simulink model "MultirotorSimPx4v1_8RateTuning"  (R2018b)
settings: Solver=VariableStepAuto  StartTime=0.0  StopTime=Simulation.T_END  MaxStep=Simulation.TS_MAX  RelTol=1e-3  EnableMultiTasking=on
PreLoadFcn:
  | % InitializeParameters;
undefined symbols (not defined in the file): Initial, Simulation, Uav
libraries: QuaternionLibrary x13, simulink_extras x10
(part 1 of 7)
settings Model: Creator=jban039  LastModifiedBy=jban039
settings DataIOCC: Decimation=10  ReturnWorkspaceOutputs=on  OutputOption=SpecifiedOutputTimes  OutputTimes=Simulation.T_OUT
settings OptimizationCC: LifeSpan=inf
settings DebuggingCC: ReadBeforeWriteMsg=DisableAll  WriteAfterWriteMsg=DisableAll  WriteAfterReadMsg=DisableAll  MultiTaskDSMMsg=none  UnconnectedLineMsg=none  AllowSymbolicDim=off  SFUnexpectedBacktrackingDiag=warning  SFNoUnconditionalDefaultTransitionDiag=warning  SFExecutionAtInitializationDiag=none  UnderSpecifiedDimensionMsg=warning
settings ModelReferenceCC: UpdateModelReferenceTargets=IfOutOfDate  ModelReferenceMinAlgLoopOccurrences=on  PropagateSignalLabelsOutOfModel=off
settings SFSimCC: SFSimEcho=off  SimUseLocalCustomCode=off
settings RTWCC: RTWUseLocalCustomCode=off
settings CodeAppCC: StateflowObjectComments=on
settings GRTTargetCC: TargetLangStandard=C89/C90 (ANSI)
settings ConfigComp: CovMetricSettings=dw  CovHtmlReporting=on  CovSaveCumulativeToWorkspaceVar=on  CovSaveSingleToWorkspaceVar=on  CovExternalEMLEnable=off

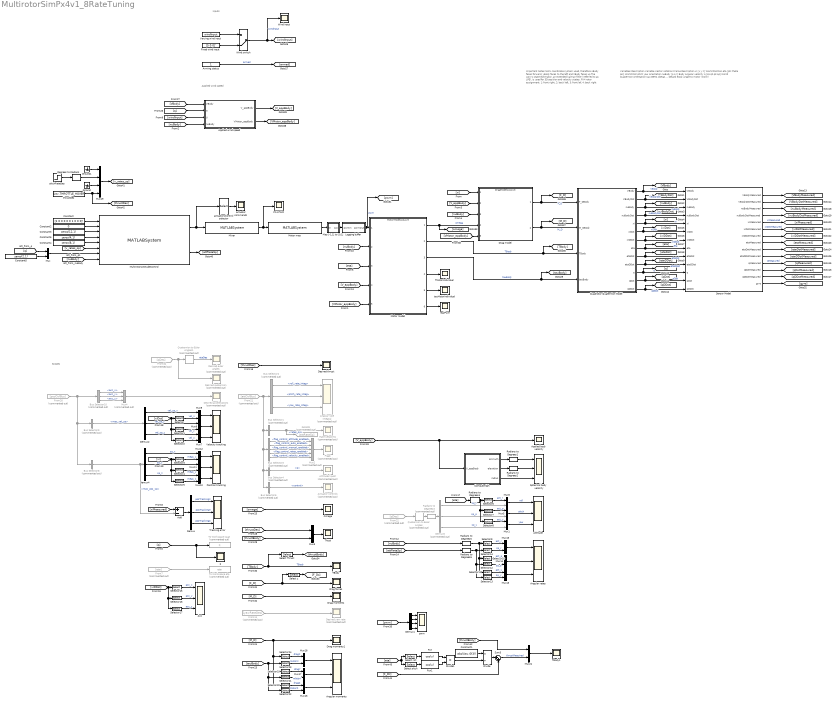
== system MultirotorSimPx4v1_8RateTuning ==
  note: Important Notes
      |
      | NWU coordinate system used, therefore xBody faces forward, yBody faces to the left and zBody faces up
      | The UAV's state estimator, an extended kalman filter (referred to as LPE), is used for 3D position and velocity states.
      | PX4 rotor assignment: 1: front right, 2: back left, 3: front lef, 4: back right
  note: Variables Description
      |
      | Variable
      | Vector notation
      | Frame
      | Description
      |
      | xi
      | [x y z]
      | World
      | Position
      |
      | eta
      | [phi theta psi]
      | World
      | Roll pitch yaw orientation
      |
      | nuBody
      | [p q r]
      | Body
      | Angular velocity
      |
      | q
      | [q1 q2 q3 q4]
      | World
      | Quaternion orientation
      |
      | Uav.BETA
      | [beta1 ... betaN]
      | Body
      | Angle to motor (CCW)
  note: Applied wind speed
  note: Inputs
  note: Scopes
  Acc : Scope  NumInputPorts=3
  Actuator controls : Scope  Commented=on
  Add : Sum  Inputs=+-
  Angular moments : Scope  NumInputPorts=3
  Angular rate integral : Scope  Commented=on  NumInputPorts=3
  Angular rates : Scope  NumInputPorts=3
  Applied body velocity : Scope
  Applied wind speed : Subsystem
  Arming status : Constant
  Attitude : Scope  NumInputPorts=3
  Attitude (quat) : Scope  Commented=on
  Bus Selector1 : BusSelector  Commented=on  OutputSignals=rates_sp
  Bus Selector10 : BusSelector  Commented=on  OutputSignals=mpc_local_pos_sp.acc_x,mpc_local_pos_sp.acc_y,mpc_local_pos_sp.acc_z
  Bus Selector2 : BusSelector  Commented=on  OutputSignals=controller_status.roll_rate_integ,controller_status.pitch_rate_integ,controller_status.yaw_rate_integ
  Bus Selector3 : BusSelector  Commented=on  OutputSignals=v_control_mode.flag_control_attitude_enabled,v_control_mode.flag_control_auto_enabled,v_control_mode.flag_control_manual_enabled,v_control_mode.flag_control_rates_enabled,v_control_mode.flag_control_velocity_enabled
  Bus Selector4 : BusSelector  Commented=on  OutputSignals=ctrl_state.q
  Bus Selector6 : BusSelector  Commented=on  OutputSignals=actuators.control
  Bus Selector8 : BusSelector  Commented=on  OutputSignals=mpc_pos_sp
  Bus Selector9 : BusSelector  Commented=on  OutputSignals=mpc_vel_sp
  Compute Sph : MATLAB Function  TreatAsAtomicUnit=on
  Constant : Constant  Value=[1 0 0 0 0 0 1 0 0 0]'
  Constant1 : Constant  Value=abs(Uav.G(3))
  Constant2 : Constant  Value=0
  Constant3 : Constant  Value=zeros(12,1)
  Constant4 : Constant  Value=zeros(8,1)
  Constant5 : Constant  Value=zeros(2,1)
  Constant6 : Constant  Value=zeros(4,1)
  Degrees to Radians : simulink_extras/Transformations/Degrees to Radians
  Demux : Demux  Outputs=3
  Demux1 : Demux
  Demux2 : Demux  Outputs=3
  Demux4 : Demux  Outputs=3
  Demux6 : Demux  Commented=on  Outputs=3
  Desired accelerations : Scope  Commented=on
  Desired euler angles : Scope  Commented=on
  Desired quaternion : Scope  Commented=on
  Desired thrust : Scope
  Desired yaw rate : Scope  Commented=on
  Divide : Product  Inputs=*/
  Divide1 : Product  Inputs=**
  Drag forces : Scope
  Drag model : ModelReference  ModelNameDialog=DragModelAIAAv3  SimulationMode=Normal  ModelReferenceVersion=1.368
  Drag moments : Scope
  Drag moments1 : Scope
  Fcn : Fcn  Expr=cos(u)
  Fcn1 : Fcn  Expr=cos(u)
  Fixed wind input : Constant  Value=[5 0 0]'
  Flags : Scope  Commented=on
  From11 : From  Commented=on  GotoTag=yawRateDes
  From20 : From  Commented=on  GotoTag=posCtrlBus
  From21 : From  Commented=on  GotoTag=attCtrlBus
  From22 : From  Commented=on  GotoTag=qDes
  From34 : From  Commented=on  GotoTag=qDes
  From7 : From  Commented=on  GotoTag=eta
  Goto28 : Goto  Commented=on  GotoTag=attRateSp
  Ground : Ground
  Ground1 : Ground
  Logging buffer : Subsystem
  Map [-1,1] to [0,1] : Subsystem
  Mixer : MATLABSystem  System=MultirotorMixer  airframeConfig=5  useHorThrust=0  outputSatStatus=0  SimulateUsing=Code generation
      mask Type: MultirotorMixer
      mask Display:
      | disp(['MULTIROTOR' char(10) 'MIXER' char(10) 'octa_x']);
      | port_label('input',1,'actuatorsControl');
      | port_label('output',1,'px4PWM');
  Motor map : MATLABSystem  System=MotorMap  airframeConfig=5  SimulateUsing=Code generation
      mask Type: MotorMap
      mask Display:
      | disp(['MOTOR' char(10) 'MAP' char(10) 'octa_x']);
      | port_label('input',1,'px4PWM');
      | port_label('output',1,'simPWM');
  Motor model : ModelReference  ModelNameDialog=MotorModelAIAAv3  SimulationMode=Normal  ModelReferenceVersion=1.397
  MultirotorAttitudeControl : MATLABSystem  System=MulticopterAttitudeControl  acro_expo_rp=0.69  acro_expo_y=0.69  acro_pitch_max=720  acro_roll_max=720  acro_superexpo_rp=0.7  acro_superexpo_y=0.7  acro_yaw_max=540  airmode=0  d_term_cutoff_freq=30  pitch_rate_d=0.003  pitch_rate_ff=0  pitch_rate_i=0.05  pitch_rate_max=220  pitch_rate_p=0.15  pitch_p=6.5  pitch_rate_integ_lim=0.3  rattitude_thres=0.8  roll_rate_d=0.003  roll_rate_ff=0  roll_rate_i=0.05  roll_rate_max=220  roll_rate_p=0.15  roll_p=6.5  roll_rate_integ_lim=0.3  tpa_breakpoint_d=1  tpa_breakpoint_i=1  tpa_breakpoint_p=1  tpa_rate_d=0  tpa_rate_i=0  tpa_rate_p=0  yaw_rate_d=0  yaw_rate_ff=0  yaw_rate_i=0.1  yaw_rate_max=200  yaw_rate_p=0.2  yaw_auto_max=45  yaw_p=2.8  yaw_rate_integ_lim=0.3  man_throttle_min=0.08  man_tilt_max_deg=35  yaw_rate_scaling=200  throttle_hover=0.5  throttle_max=1  board_rotation_param=0  board_offset_x=0  board_offset_y=0  board_offset_z=0  bat_scale_en=0  throttle_curve=0  vehicle_status_is_rotary_wing=1  vehicle_status_is_vtol=0  loop_update_rate_hz=250  simple_mode=0  output_rates=1  SimulateUsing=Code generation
      mask Type: MulticopterAttitudeControl
      mask Display:
      | disp(['MulticopterAttitudeControl' char(10) '' char(10) 'v1.82']);
      | port_label('input',1,'v_control_mode_flags');
      | port_label('input',2,'vehicle_land_detected');
      | port_label('input',3,'saturation_status');
      | port_label('input',4,'manual_control_sp');
      | port_label('input',5,'v_att_sp');
      | port_label('input',6,'v_rates_sp');
      | port_label('input',7,'v_att_in');
      | port_label('input',8,'sensor_gyro');
      | port_label('output',1,'actuatorsControl');
      | port_label('output',2,'attRateSp');
  Mux{,1,3,5..18,21} (18 alike) : Mux  Inputs=2
  Mux19 : Mux
  Mux2 : Mux  Commented=on  Inputs=5
  Mux4 : Mux  Commented=on  Inputs=3
  Omega : Scope
  PX4 PWM : Scope
  Position tracking : Scope  NumInputPorts=3
  Quadrotor Quaternion Model : Subsystem
  Quaternion to Euler Angles : QuaternionLibrary/Quaternion to Euler Angles  Commented=on
  Quaternion to Euler Angles1 : QuaternionLibrary/Quaternion to Euler Angles  Commented=on
  Radians to Degrees{1..2,4..6} (5 alike) : simulink_extras/Transformations/Radians to Degrees
  Radians to Degrees3 : simulink_extras/Transformations/Radians to Degrees  Commented=on
  Rate setpoints : Scope  Commented=on
  Select Thrust : Selector  InputPortWidth=3  IndexOptions=Index vector (dialog)  Indices=[3]  OutputSizes=1
  Select pitch : Selector  InputPortWidth=3  IndexOptions=Index vector (dialog)  Indices=2  OutputSizes=1
  Select roll : Selector  InputPortWidth=3  IndexOptions=Index vector (dialog)  Indices=1  OutputSizes=1
  Select z : Selector  InputPortWidth=3  IndexOptions=Index vector (dialog)  Indices=[3]  OutputSizes=1
  Selector{,3,6,9,14..15,23..24} (8 alike) : Selector  InputPortWidth=3  IndexOptions=Index vector (dialog)  Indices=1  OutputSizes=1
  Selector{1,4,7,10,12,16,19,21} (8 alike) : Selector  InputPortWidth=3  IndexOptions=Index vector (dialog)  Indices=2  OutputSizes=1
  Selector{2,5,8,11,13,17,20,22} (8 alike) : Selector  InputPortWidth=3  IndexOptions=Index vector (dialog)  Indices=3  OutputSizes=1
  Sensor Model : Subsystem
  Spherical body velocity : Scope  NumInputPorts=3
  Sum3 : Sum  Inputs=|++
  TBody : Scope
  TBody1 : Scope
  TMotorIndividual : Scope
  Thust : Scope
  To Workspace eta : ToWorkspace  Commented=on  VariableName=eta  SaveFormat=Structure With Time  SampleTime=0.01
  To Workspace quat : ToWorkspace  Commented=on  VariableName=q  SaveFormat=Structure With Time  SampleTime=0.01
  Tracking error : Scope  NumInputPorts=3
  Varying wind input : FromWorkspace  VariableName=windInput  SampleTime=0
  Velocity tracking : Scope  NumInputPorts=3
  Wind Input : Scope
  Wind switch : ManualSwitch  CurrentSetting=0
  actuator commands : Scope
  actuatorsControl selector : Selector  InputPortWidth=8  IndexOptions=Index vector (dialog)  Indices=[1 2 3]  OutputSizes=1
  pitchRateDes : Step  After=30  SampleTime=0
  pwm : Scope  NumInputPorts=4
  q : Scope
  realPwm : Scope
  tauMotorIndividual : Scope
  thrustDes : Constant  Value=Uav.THROTTLE_HOVER
  wires:
  Motor model/1 -> [omega], Drag model/4  "omega"
  Motor model/2 -> Quadrotor Quaternion Model/3(TBody), [TBody]  "TBody"
  Drag model/2 -> Quadrotor Quaternion Model/2(M_DBody), [M_D]  "M_D"
  Quadrotor Quaternion Model/1(VBody) -> Sensor Model/1(VBody), [VBody]  "VBody"
  Quadrotor Quaternion Model/2(VBodyDot) -> Sensor Model/2(VBodyDot), [VBodyDot]  "VBodyDot"
  Quadrotor Quaternion Model/3(nuBody) -> Sensor Model/3(nuBody), [nuBody]  "nuBody"
  Quadrotor Quaternion Model/4(nuBodyDot) -> Sensor Model/4(nuBodyDot), [nuBodyDot]  "nuBodyDot"
  Quadrotor Quaternion Model/5(xi) -> Sensor Model/5(xi), [xi]  "xi"
  Quadrotor Quaternion Model/6(xiDot) -> Sensor Model/6(xiDot), [xiDot]  "xiDot"
  Quadrotor Quaternion Model/7(xiDDot) -> Sensor Model/7(xiDDot), [xiDDot]  "xiDDot"
  Quadrotor Quaternion Model/8(eta) -> Sensor Model/8(eta), [eta]  "eta"
  Quadrotor Quaternion Model/9(etaDot) -> Sensor Model/9(etaDot), [etaDot]  "etaDot"
  Quadrotor Quaternion Model/10(etaDDot) -> Sensor Model/10(etaDDot), [etaDDot]  "etaDDot"
  [V_appBody] -> Drag model/2
  [nuBody] -> Motor model/2
  Quadrotor Quaternion Model/11(q) -> Sensor Model/11(q), [q]  "q"
  Quadrotor Quaternion Model/12(qDot) -> Sensor Model/12(qDot), [qDot]  "qDot"
  Quadrotor Quaternion Model/13(qDDot) -> Sensor Model/13(qDDot), [qDDot]  "qDDot"
  Drag model/1 -> Quadrotor Quaternion Model/1(F_DBody), [F_D]  "F_D"
  Sensor Model/1(VBodyMeasured) -> [VBodyMeasured]
  Sensor Model/2(VBodyDotMeasured) -> [VBodyDotMeasured]
  Sensor Model/3(nuBodyMeasured) -> [nuBodyMeasured]
  Sensor Model/4(nuBodyDotMeasured) -> [nuBodyDotMeasured]
  Sensor Model/5(xiMeasured) -> [xiMeasured]  "xiMeasured"
  Sensor Model/6(xiDotMeasured) -> [xiDotMeasured]  "xiDotMeasured"
  Sensor Model/7(xiDDotMeasured) -> [xiDDotMeasured]
  Sensor Model/8(etaMeasured) -> [etaMeasured]
  Sensor Model/9(etaDotMeasured) -> [etaDotMeasured]
  Sensor Model/10(etaDDotMeasured) -> [etaDDotMeasured]
  Sensor Model/11(qMeasured) -> [qMeasured]  "qMeasured"
  Sensor Model/12(qDotMeasured) -> [qDotMeasured]
  Sensor Model/13(qDDotMeasured) -> [qDDotMeasured]
  Logging buffer/1(pwmOut) -> [pwm], Motor model/1  "pwm"
  Bus Selector2/1 -> Angular rate integral/1  "<roll_rate_integ>"
  Bus Selector2/2 -> Angular rate integral/2  "<pitch_rate_integ>"
  Bus Selector2/3 -> Angular rate integral/3  "<yaw_rate_integ>"
  From21/1 -> Bus Selector2/1, Bus Selector1/1, Bus Selector6/1, Bus Selector4/1, Bus Selector3/1
  Bus Selector1/1 -> Goto28/1, Rate setpoints/1  "<rates_sp>"
  Bus Selector3/1 -> Mux2/1  "<flag_control_attitude_enabled>"
  Bus Selector3/2 -> Mux2/2  "<flag_control_auto_enabled>"
  Bus Selector3/3 -> Mux2/3  "<flag_control_manual_enabled>"
  Bus Selector3/4 -> Mux2/4  "<flag_control_rates_enabled>"
  Bus Selector3/5 -> Mux2/5  "<flag_control_velocity_enabled>"
  Mux2/1 -> Flags/1
  Bus Selector4/1 -> Attitude (quat)/1  "<q>"
  Bus Selector6/1 -> Actuator controls/1  "<control>"
  From20/1 -> Bus Selector10/1, Bus Selector9/1, Bus Selector8/1
  [q] -> Mux/1
  Bus Selector9/1 -> Demux2/1  "<mpc_vel_sp>"
  Bus Selector10/1 -> Mux4/1  "<acc_x>"
  Bus Selector10/2 -> Mux4/2  "<acc_y>"
  Bus Selector10/3 -> Mux4/3  "<acc_z>"
  Mux4/1 -> Desired accelerations/1
  Selector6/1 -> Mux6/1  "act_r"
  Selector7/1 -> Mux5/1  "act_p"
  Mux7/1 -> Velocity tracking/3
  Mux8/1 -> Velocity tracking/2
  Mux9/1 -> Velocity tracking/1
  Demux2/1 -> Mux9/1  "vel_sp_x"
  Selector/1 -> Mux9/2  "vel_x"
  Demux2/2 -> Mux8/1  "vel_sp_y"
  Selector1/1 -> Mux8/2  "vel_y"
  Demux2/3 -> Mux7/1  "vel_sp_z"
  Selector2/1 -> Mux7/2  "vel_z"
  Mux10/1 -> Position tracking/3
  Mux11/1 -> Position tracking/2
  Mux12/1 -> Position tracking/1
  Demux4/1 -> Mux12/1  "sp_x"
  Selector3/1 -> Mux12/2  "meas_x"
  Demux4/2 -> Mux11/1  "sp_y"
  Selector4/1 -> Mux11/2  "meas_y"
  Demux4/3 -> Mux10/1  "sp_z"
  Selector5/1 -> Mux10/2  "meas_z"
  Quaternion to Euler Angles/1 -> Radians to Degrees3/1
  Demux6/1 -> Mux6/2  "sp_r"
  Demux6/2 -> Mux5/2  "sp_p"
  Demux6/3 -> Mux1/2  "sp_y"
  Selector8/1 -> Mux1/1  "act_y"
  From22/1 -> Quaternion to Euler Angles/1
  Mixer/1 -> Motor map/1, PX4 PWM/1
  Bus Selector8/1 -> Add/2, Demux4/1  "<mpc_pos_sp>"
  Add/1 -> Demux/1
  Demux/1 -> Tracking error/1  "posTrackingX"
  Demux/2 -> Tracking error/2  "posTrackingY"
  Demux/3 -> Tracking error/3  "posTrackingZ"
  [nuBody] -> Drag model/3
  Mux6/1 -> Attitude/1  "roll"
  Mux5/1 -> Attitude/2  "pitch"
  [eta] -> Motor model/3
  [q] -> q/1, To Workspace quat/1
  From7/1 -> To Workspace eta/1
  [xiDot] -> Selector2/1, Selector1/1, Selector/1
  [xi] -> Selector5/1, Selector4/1, Selector3/1
  [xiMeasured] -> Add/1
  Wind switch/1 -> [windInput], Wind Input/1  "windInput"
  [V_appBody] -> Motor model/4
  Arming status/1 -> [armed]  "armed"
  Fixed wind input/1 -> Wind switch/2
  Varying wind input/1 -> Wind switch/1
  [omega] -> Omega/1
  Radians to Degrees3/1 -> Demux6/1
  Radians to Degrees4/1 -> Selector8/1, Selector7/1, Selector6/1
  [eta] -> Radians to Degrees4/1
  Motor model/4 -> TMotorIndividual/1
  [thrustDes] -> Mux3/1
  [thrustBody] -> Mux3/2
  Mux3/1 -> Thust/1
  Motor model/5 -> tauMotorIndividual/1
  [xi] -> Drag model/1
  [TBody] -> Select Thrust/1, TBody/1  "TBody"
  Select Thrust/1 -> [thrustBody]
  [F_D] -> Drag forces/1, Select z/1
  [V_appBody] -> Compute Sph/1(V_appBody), Applied body velocity/1
  Compute Sph/1(azimuth) -> Radians to Degrees1/1
  Compute Sph/2(elevation) -> Radians to Degrees2/1
  Compute Sph/3(radius) -> Spherical body velocity/3
  Radians to Degrees1/1 -> Spherical body velocity/1
  Radians to Degrees2/1 -> Spherical body velocity/2
  [M_D] -> Drag moments/1
  [VMotor_appBody] -> Motor model/5
  [VMotor_appBody] -> Drag model/5
  From11/1 -> Desired yaw rate/1
  Mux1/1 -> Attitude/3  "yaw"
  Motor model/3 -> Quadrotor Quaternion Model/4(tauBody), [tauBody]  "tauBody"
  [VBody] -> Applied wind speed/1(VBody)
  [q] -> Applied wind speed/2(q)
  [windInput] -> Applied wind speed/3(U)
  Applied wind speed/1(V_appBody) -> [V_appBody]
  Applied wind speed/2(VMotor_appBody) -> [VMotor_appBody]
  [nuBody] -> Applied wind speed/4(nuBody)
  Selector9/1 -> Mux15/1  "act_r"
  Selector10/1 -> Mux14/1  "act_p"
  Selector11/1 -> Mux13/1  "act_y"
  Mux15/1 -> Angular rates/1
  Mux14/1 -> Angular rates/2
  Radians to Degrees5/1 -> Selector9/1, Selector11/1, Selector10/1
  [nuBody] -> Radians to Degrees5/1
  Mux13/1 -> Angular rates/3
  Radians to Degrees6/1 -> Selector14/1, Selector13/1, Selector12/1
  Selector14/1 -> Mux15/2  "sp_r"
  Selector12/1 -> Mux14/2  "sp_p"
  Selector13/1 -> Mux13/2  "sp_y"
  [attRateSp] -> Radians to Degrees6/1
  Selector15/1 -> Acc/1  "acc_x"
  Selector16/1 -> Acc/2  "acc_y"
  Selector17/1 -> Acc/3  "acc_z"
  [xiDDot] -> Selector15/1, Selector16/1, Selector17/1
  [thrustDes] -> Desired thrust/1
  actuatorsControl selector/1 -> actuator commands/1
  [M_D] -> Selector20/1, Selector19/1, Selector24/1, Drag moments1/1
  Mux18/1 -> Angular moments/1
  Mux17/1 -> Angular moments/2
  Mux16/1 -> Angular moments/3
  Selector24/1 -> Mux18/1  "dragX"
  Selector23/1 -> Mux18/2  "motorX"
  Selector19/1 -> Mux17/1  "dragY"
  Selector21/1 -> Mux17/2  "motorY"
  Selector20/1 -> Mux16/1  "dragZ"
  Selector22/1 -> Mux16/2  "MotorZ"
  [tauBody] -> Selector22/1, Selector21/1, Selector23/1
  From34/1 -> Desired quaternion/1, Quaternion to Euler Angles1/1
  Quaternion to Euler Angles1/1 -> Desired euler angles/1  "etaDes"
  Divide/1 -> Sum3/1
  Sum3/1 -> Mux21/2  "thrustRequired"
  Mux21/1 -> TBody1/1
  Constant1/1 -> Divide/1
  Select z/1 -> [F_Dz]
  [thrustBody] -> Mux21/1
  [eta] -> Select pitch/1, Select roll/1
  Select roll/1 -> Fcn/1
  Select pitch/1 -> Fcn1/1
  Fcn/1 -> Divide1/1
  Fcn1/1 -> Divide1/2
  Divide1/1 -> Divide/2
  [F_Dz] -> Sum3/2
  [pwm] -> Demux1/1
  Demux1/1 -> pwm/1
  Demux1/2 -> pwm/2
  Demux1/3 -> pwm/3
  Demux1/4 -> pwm/4
  Motor model/6 -> realPwm/1
  Sensor Model/14(gyro) -> [gyro]
  [nuBody] -> MultirotorAttitudeControl/8
  MultirotorAttitudeControl/2 -> [attRateSp]
  Motor map/1 -> Map [-1,1] to [0,1]/1(in)
  Map [-1,1] to [0,1]/1(out) -> Logging buffer/1(pwmIn)
  MultirotorAttitudeControl/1 -> Mixer/1, actuatorsControl selector/1
  Constant/1 -> MultirotorAttitudeControl/1
  Constant2/1 -> MultirotorAttitudeControl/2
  Constant3/1 -> MultirotorAttitudeControl/3
  Constant4/1 -> MultirotorAttitudeControl/5
  Constant5/1 -> Mux/2
  Mux/1 -> MultirotorAttitudeControl/7
  Constant6/1 -> MultirotorAttitudeControl/4
  [v_rates_sp] -> MultirotorAttitudeControl/6
  Mux19/1 -> [v_rates_sp]
  pitchRateDes/1 -> Degrees to Radians/1
  Ground/1 -> Mux19/3
  thrustDes/1 -> [thrustDes], Mux19/4
  Ground1/1 -> Mux19/1
  Degrees to Radians/1 -> Mux19/2

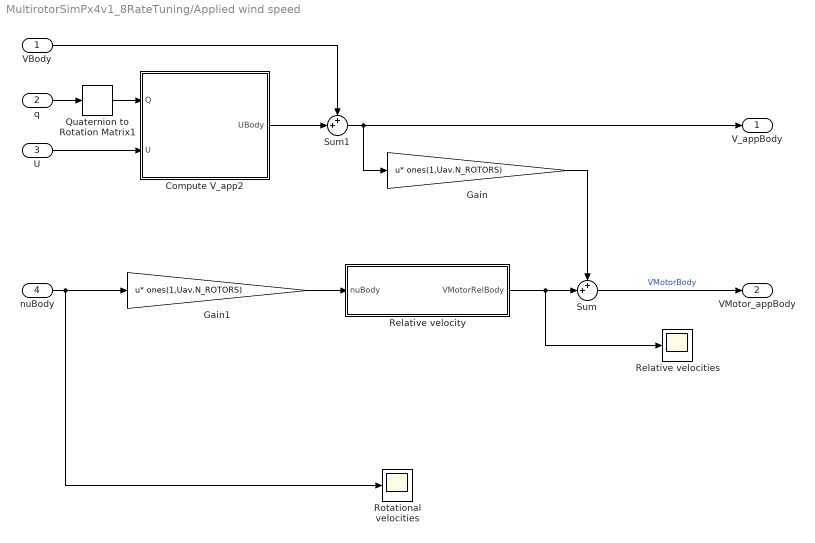
== system MultirotorSimPx4v1_8RateTuning/Applied wind speed ==
  VBody : Inport  Unit=m/s
  q : Inport  Port=2
  U : Inport  Port=3  Unit=m/s
  nuBody : Inport  Port=4  Unit=rad/s
  Compute V_app2 : MATLAB Function  TreatAsAtomicUnit=on
  Gain : Gain  Gain=ones(1,Uav.N_ROTORS)  Multiplication=Matrix(u*K)
  Gain1 : Gain  Gain=ones(1,Uav.N_ROTORS)  Multiplication=Matrix(u*K)
  Quaternion to Rotation Matrix1 : QuaternionLibrary/Quaternion to Rotation Matrix
  Relative velocities : Scope
  Relative velocity : MATLAB Function  TreatAsAtomicUnit=on
  Rotational velocities : Scope
  Sum : Sum  Inputs=++|
  Sum1 : Sum  Inputs=++|
  V_appBody : Outport  Unit=m/s
  VMotor_appBody : Outport  Port=2  Unit=m/s  PortDimensions=[3,Uav.N_ROTORS]
  wires:
  U/1 -> Compute V_app2/2(U)
  Sum/1 -> VMotor_appBody/1  "VMotorBody"
  Quaternion to Rotation Matrix1/1 -> Compute V_app2/1(Q)
  nuBody/1 -> Gain1/1, Rotational velocities/1
  Gain/1 -> Sum/1
  VBody/1 -> Sum1/1
  q/1 -> Quaternion to Rotation Matrix1/1
  Relative velocity/1(VMotorRelBody) -> Relative velocities/1, Sum/2
  Compute V_app2/1(UBody) -> Sum1/2
  Sum1/1 -> Gain/1, V_appBody/1
  Gain1/1 -> Relative velocity/1(nuBody)

== system MultirotorSimPx4v1_8RateTuning/Logging buffer ==
  pwmIn : Inport
  Rate Transition : RateTransition
  pwmOut : Outport
  wires:
  pwmIn/1 -> Rate Transition/1
  Rate Transition/1 -> pwmOut/1

== system MultirotorSimPx4v1_8RateTuning/Map [-1,1] to [0,1] ==
  in : Inport
  Constant : Constant
  Gain4 : Gain  Gain=0.5
  Sum : Sum  Inputs=++|
  out : Outport
  wires:
  Sum/1 -> Gain4/1
  Gain4/1 -> out/1
  in/1 -> Sum/2
  Constant/1 -> Sum/1

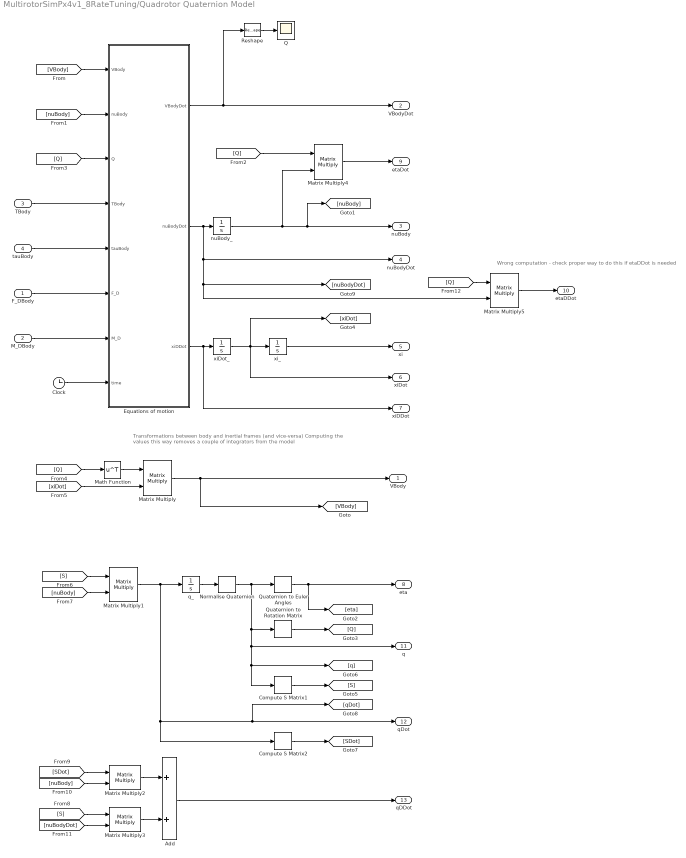
== system MultirotorSimPx4v1_8RateTuning/Quadrotor Quaternion Model ==
  note: Wrong computation - check proper way to do this if etaDDot is needed
  note: Transformations between body and inertial frames (and vice-versa)
      | Computing the values this way removes a couple of integrators from the model
  F_DBody : Inport  Unit=N
  M_DBody : Inport  Port=2  Unit=N*m
  TBody : Inport  Port=3  Unit=N
  tauBody : Inport  Port=4  Unit=N*m
  Add : Sum
  Clock : Clock
  Compute S Matrix1 : QuaternionLibrary/Compute S Matrix
  Compute S Matrix2 : QuaternionLibrary/Compute S Matrix
  Equations of motion : MATLAB Function  TreatAsAtomicUnit=on
  Math Function : Math  Operator=transpose  SaturateOnIntegerOverflow=on
  Matrix Multiply{,1..5} (6 alike) : Product  Multiplication=Matrix(*)
  Normalise Quaternion : QuaternionLibrary/Normalise Quaternion
  Q : Scope
  Quaternion to Euler Angles : QuaternionLibrary/Quaternion to Euler Angles
  Quaternion to Rotation Matrix : QuaternionLibrary/Quaternion to Rotation Matrix
  Reshape : Reshape  OutputDimensionality=Column vector (2-D)
  nuBody_ : Integrator  InitialCondition=Initial.NU_BODY  ContinuousStateAttributes='nuBody'
  q_ : Integrator  InitialCondition=Initial.Q  ContinuousStateAttributes='q'
  xiDot_ : Integrator  InitialCondition=Initial.XI_DOT  ContinuousStateAttributes='xiDot'
  xi_ : Integrator  InitialCondition=Initial.XI  ContinuousStateAttributes='xi'
  VBody : Outport  Unit=m/s
  VBodyDot : Outport  Port=2  Unit=m/s^2
  nuBody : Outport  Port=3  Unit=rad/s
  nuBodyDot : Outport  Port=4  Unit=rad/s^2
  xi : Outport  Port=5  Unit=m
  xiDot : Outport  Port=6  Unit=m/s
  xiDDot : Outport  Port=7  Unit=m/s^2
  eta : Outport  Port=8  Unit=rad
  etaDot : Outport  Port=9  Unit=rad/s
  etaDDot : Outport  Port=10  Unit=rad/s^2
  q : Outport  Port=11
  qDot : Outport  Port=12
  qDDot : Outport  Port=13
  wires:
  Equations of motion/1(VBodyDot) -> Reshape/1, VBodyDot/1
  xi_/1 -> xi/1
  [nuBody] -> Equations of motion/2(nuBody)
  [VBody] -> Equations of motion/1(VBody)
  tauBody/1 -> Equations of motion/5(tauBody)
  TBody/1 -> Equations of motion/4(TBody)
  Equations of motion/3(xiDDot) -> xiDot_/1, xiDDot/1
  F_DBody/1 -> Equations of motion/6(F_D)
  Matrix Multiply/1 -> VBody/1, [VBody]
  M_DBody/1 -> Equations of motion/7(M_D)
  nuBody_/1 -> Matrix Multiply4/2, [nuBody], nuBody/1
  Equations of motion/2(nuBodyDot) -> nuBody_/1, nuBodyDot/1, Matrix Multiply5/2, [nuBodyDot]
  q_/1 -> Normalise Quaternion/1
  Quaternion to Euler Angles/1 -> eta/1, [eta]
  Matrix Multiply4/1 -> etaDot/1
  Quaternion to Rotation Matrix/1 -> [Q]
  [Q] -> Equations of motion/3(Q)
  [Q] -> Math Function/1
  [xiDot] -> Matrix Multiply/2
  Math Function/1 -> Matrix Multiply/1
  [S] -> Matrix Multiply1/1
  [nuBody] -> Matrix Multiply1/2
  Compute S Matrix2/1 -> [SDot]
  [S] -> Matrix Multiply3/1
  Matrix Multiply1/1 -> qDot/1, [qDot], Compute S Matrix2/1, q_/1
  [SDot] -> Matrix Multiply2/1
  [nuBody] -> Matrix Multiply2/2
  [nuBodyDot] -> Matrix Multiply3/2
  Matrix Multiply2/1 -> Add/1
  Matrix Multiply3/1 -> Add/2
  Normalise Quaternion/1 -> Quaternion to Euler Angles/1, q/1, Compute S Matrix1/1, [q], Quaternion to Rotation Matrix/1
  Compute S Matrix1/1 -> [S]
  [Q] -> Matrix Multiply4/1
  Add/1 -> qDDot/1
  [Q] -> Matrix Multiply5/1
  Matrix Multiply5/1 -> etaDDot/1
  Reshape/1 -> Q/1
  xiDot_/1 -> xi_/1, [xiDot], xiDot/1
  Clock/1 -> Equations of motion/8(time)

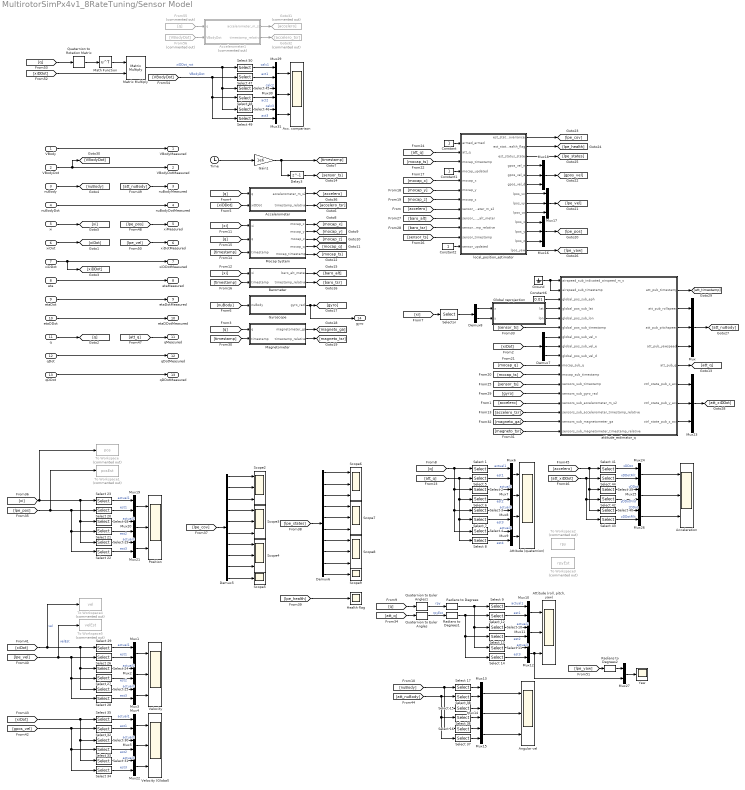
== system MultirotorSimPx4v1_8RateTuning/Sensor Model ==
  VBody : Inport  Unit=m/s  PortDimensions=3
  VBodyDot : Inport  Port=2  Unit=m/s^2  PortDimensions=3
  nuBody : Inport  Port=3  Unit=rad/s  PortDimensions=3
  nuBodyDot : Inport  Port=4  Unit=rad/s^2  PortDimensions=3
  xi : Inport  Port=5  Unit=m  PortDimensions=3
  xiDot : Inport  Port=6  Unit=m/s  PortDimensions=3
  xiDDot : Inport  Port=7  Unit=m/s^2  PortDimensions=3
  eta : Inport  Port=8  Unit=rad  PortDimensions=3
  etaDot : Inport  Port=9  Unit=rad/s  PortDimensions=3
  etaDDot : Inport  Port=10  Unit=rad/s^2  PortDimensions=3
  q : Inport  Port=11  PortDimensions=4
  qDot : Inport  Port=12  PortDimensions=4
  qDDot : Inport  Port=13  PortDimensions=4
  Acc. comparison : Scope  NumInputPorts=3
  Acceleration : Scope  NumInputPorts=3
  Accelerometer : Subsystem
  Accelerometer1 : Subsystem  Commented=on
  Angular vel : Scope  NumInputPorts=3
  Attitude (quaternion) : Scope  NumInputPorts=4
  "Attitude (roll, pitch, yaw)" : Scope  NumInputPorts=3
  Barometer : Subsystem
  Constant : Constant
  Constant1 : Constant
  Constant2 : Constant
  Constant6 : Constant  Value=0.01
  Delay3 : Delay  DelayLength=1  SampleTime=1/400  StateName=sensorTs
  Demux5 : Demux  Outputs=10
  Demux6 : Demux  Outputs=10
  Demux7 : Demux  Outputs=3
  Demux8 : Demux  Outputs=2
  From55 : From  Commented=on  GotoTag=q
  From56 : From  Commented=on  GotoTag=VBodyDot
  Gain1 : Gain  Gain=1e6
  Global reprojection : Subsystem  AncestorBlock=Px4Library/Global reprojection  mask{LAT0=-36.865577, LON0=174.772065}
      mask prompts: LAT0 "Latitude at [x,y] = [0,0]"; LON0 "Longitude at [x,y] = [0,0]"
      mask Display:
      | disp('REPROJECT')
      | port_label('input', 1, sprintf('x'))
      | port_label('input', 2, sprintf('y'))
      | port_label('output', 1, sprintf('lat'))
      | port_label('output', 2, sprintf('lon'))
  Goto31 : Goto  Commented=on  GotoTag=accelero
  Goto32 : Goto  Commented=on  GotoTag=accelero_tsr
  Ground : Ground
  Gyroscope : Subsystem
  Health flag : Scope
  Magnetometer : Subsystem
  Math Function : Math  Operator=transpose  SaturateOnIntegerOverflow=on
  Matrix Multiply : Product  Multiplication=Matrix(*)
  Mocap System : Subsystem
  Mux{,16..18,23} (5 alike) : Mux  Inputs=3
  Mux{1..15,19..22,24..27,29..31} (26 alike) : Mux  Inputs=2
  Position : Scope  NumInputPorts=3
  Quaternion to Euler Angles : QuaternionLibrary/Quaternion to Euler Angles
  Quaternion to Euler Angles1 : QuaternionLibrary/Quaternion to Euler Angles
  Quaternion to Rotation Matrix : QuaternionLibrary/Quaternion to Rotation Matrix
  Radians to Degrees : simulink_extras/Transformations/Radians to Degrees
  Radians to Degrees1 : simulink_extras/Transformations/Radians to Degrees
  Radians to Degrees2 : simulink_extras/Transformations/Radians to Degrees
  Scope{2..4,6..8} (6 alike) : Scope  NumInputPorts=3
  Scope5 : Scope
  Scope9 : Scope
  Select 1 : Selector  InputPortWidth=4  IndexOptions=Index vector (dialog)  Indices=1  OutputSizes=1
  Select {10,13,15,18,21,24,27,30,33,36,39,42,45,48} (14 alike) : Selector  InputPortWidth=3  IndexOptions=Index vector (dialog)  Indices=2  OutputSizes=1
  Select {11,14,16,19,22,25,28,31,34,37,40,43,46,49} (14 alike) : Selector  InputPortWidth=3  IndexOptions=Index vector (dialog)  Indices=3  OutputSizes=1
  Select {9,12,17,20,23,26,29,32,35,38,41,44,47,50} (14 alike) : Selector  InputPortWidth=3  IndexOptions=Index vector (dialog)  Indices=1  OutputSizes=1
  Select 2 : Selector  InputPortWidth=4  IndexOptions=Index vector (dialog)  Indices=2  OutputSizes=1
  Select 3 : Selector  InputPortWidth=4  IndexOptions=Index vector (dialog)  Indices=3  OutputSizes=1
  Select 4 : Selector  InputPortWidth=4  IndexOptions=Index vector (dialog)  Indices=4  OutputSizes=1
  Select 5 : Selector  InputPortWidth=4  IndexOptions=Index vector (dialog)  Indices=1  OutputSizes=1
  Select 6 : Selector  InputPortWidth=4  IndexOptions=Index vector (dialog)  Indices=2  OutputSizes=1
  Select 7 : Selector  InputPortWidth=4  IndexOptions=Index vector (dialog)  Indices=3  OutputSizes=1
  Select 8 : Selector  InputPortWidth=4  IndexOptions=Index vector (dialog)  Indices=4  OutputSizes=1
  Selector : Selector  InputPortWidth=3  IndexOptions=Index vector (dialog)  Indices=[1 2]  OutputSizes=1
  Time : Clock
  To Workspace : ToWorkspace  Commented=on  VariableName=pos  SaveFormat=Structure With Time  SampleTime=-1
  To Workspace1 : ToWorkspace  Commented=on  VariableName=posEst  SaveFormat=Structure With Time  SampleTime=-1
  To Workspace2 : ToWorkspace  Commented=on  VariableName=rpy  SaveFormat=Structure With Time  SampleTime=-1
  To Workspace3 : ToWorkspace  Commented=on  VariableName=rpyEst  SaveFormat=Structure With Time  SampleTime=-1
  To Workspace4 : ToWorkspace  Commented=on  VariableName=vel  SaveFormat=Structure With Time  SampleTime=-1
  To Workspace5 : ToWorkspace  Commented=on  VariableName=velEst  SaveFormat=Structure With Time  SampleTime=-1
  Velocity : Scope  NumInputPorts=3
  Velocity (Global) : Scope  NumInputPorts=3
  Yaw : Scope
  attitude_estimator_q : Subsystem  AncestorBlock=Px4Library/attitude_estimator_q  mask(PX4 LPE (local position estimator): local_position_estimator){Q_SAMPLING_PERIOD=1/250, INIT_Q=[1  0  0  0], ATT_W_ACC=0.2, ATT_W_MAG=0.1, ATT_W_EXT_HDG=0.1, ATT_W_GYRO_BIAS=0.1, ATT_MAG_DECL=0.0, ATT_MAG_DECL_A=1, ATT_EXT_HDG_M=2, ATT_ACC_COMP=1, ATT_BIAS_MAX=0.05, FW_ARSP_MODE=0}
      mask prompts: Q_SAMPLING_PERIOD "Sampling period (s)"; INIT_Q "INIT_Q - Initial UAV orientation - set to 0 to let controller decide (bugged) (-)"; ATT_W_ACC "ATT_W_ACC - Complimentary filter accelerometer weight (-)"; ATT_W_MAG "ATT_W_MAG - Complimentary filter magnetometer weight (-)"; ATT_W_EXT_HDG "ATT_W_EXT_HDG - Complimentary filter external heading weight (-)"; ATT_W_GYRO_BIAS "ATT_W_GYRO_BIAS - Complimentary filter gyroscope bias weight (-)"; ATT_MAG_DECL "ATT_MAG_DECL - Magnetic declination. Not used when GPS available (deg)"; ATT_MAG_DECL_A "ATT_MAG_DECL_A - Automatic GPS based declination compensation (-)"; ATT_EXT_HDG_M "ATT_EXT_HDG_M - External heading usage mode (from Motion capture/Vision) (-), 0 None 1 Vision 2 Motion Capture"; ATT_ACC_COMP "ATT_ACC_COMP - Acceleration compensation based on GPS velocity. (-)"; ATT_BIAS_MAX "ATT_BIAS_MAX - Gyro bias limit (rad/s)"; FW_ARSP_MODE "FW_ARSP_MODE - Method used to publish the airspeed (-), 0 Measured airspeed 1 Vehicle ground speed 2 Airspeed invalid"
      mask TypeOptions ATT_EXT_HDG_M: 0 | 1 | 2
      mask TypeOptions FW_ARSP_MODE: 0 | 1 | 2
  local_position_estimator : Subsystem  AncestorBlock=Px4Library/local_position_estimator  mask(PX4 LPE (local position estimator): local_position_estimator){LPE_SAMPLING_PERIOD=0.01, LPE_ACC_XY=0.012, LPE_ACC_Z=0.02, LPE_BAR_Z=3, LPE_EPH_MAX=3, LPE_EPV_MAX=5, LPE_FAKE_ORIGIN=0, LPE_FGYRO_HP=0.001, LPE_FLW_OFF_Z=0, LPE_FLW_QMIN=150, LPE_FLW_R=7, LPE_FLW_RR=7, LPE_FLW_SCALE=1.3, LPE_GPS_DELAY=0.29, LPE_GPS_VXY=0.25, LPE_GPS_VZ=0.25, LPE_GPS_XY=1, LPE_GPS_Z=3, LPE_LAND_VXY=0.05, LPE_LAND_Z=0.03, LPE_LAT=47.3977, LPE_LDR_OFF_Z=0, LPE_LDR_Z=0.03, LPE_LON=8.5456, LPE_PN_B=0.001, LPE_PN_P=0.1, LPE_PN_T=0.001, LPE_PN_V=0.1, LPE_SNR_OFF_Z=0, LPE_SNR_Z=0.05, LPE_T_MAX_GRADE=1, LPE_VIC_P=0.001, LPE_VIS_DELAY=0.1, LPE_VIS_XY=0.1, LPE_VIS_Z=0.5, LPE_VXY_PUB=0.3, LPE_X_LP=5, LPE_Z_PUB=1, LPE_FUSION=193, Barometer=on, GPS=off, LIDAR=off, Flow=off, Sonar=off, Vision=off, Mocap=on, Land=on}
      mask prompts: LPE_SAMPLING_PERIOD "Sampling period (s)"; LPE_ACC_XY "LPE_ACC_XY - Accelerometer xy noise density (m/s^2/sqrt(Hz))"; LPE_ACC_Z "LPE_ACC_Z - Accelerometer z noise density (m/s^2/sqrt(Hz))"; LPE_BAR_Z "LPE_BAR_Z - Barometric presssure altitude z standard deviation. (m)"; LPE_EPH_MAX "LPE_EPH_MAX - Max EPH allowed for GPS initialization (m)"; LPE_EPV_MAX "LPE_EPV_MAX - Max EPV allowed for GPS initialization (m)"; LPE_FAKE_ORIGIN "LPE_FAKE_ORIGIN - Enable publishing of a fake global position (e.g for AUTO missions using Optical Flow) (-)"; LPE_FGYRO_HP "LPE_FGYRO_HP - Flow gyro high pass filter cut off frequency (Hz)"; LPE_FLW_OFF_Z "LPE_FLW_OFF_Z - Optical flow z offset from center (m)"; LPE_FLW_QMIN "LPE_FLW_QMIN - Optical flow minimum quality threshold (-)"; LPE_FLW_R "LPE_FLW_R - Optical flow rotation (roll/pitch) noise gain (m/s / (rad))"; LPE_FLW_RR "LPE_FLW_RR - Optical flow angular velocity noise gain (m/s / (rad/s))"; LPE_FLW_SCALE "LPE_FLW_SCALE - Optical flow scale (m)"; LPE_GPS_DELAY "LPE_GPS_DELAY - GPS delay compensaton (sec)"; LPE_GPS_VXY "LPE_GPS_VXY - GPS xy velocity standard deviation. (m/s)"; LPE_GPS_VZ "LPE_GPS_VZ - GPS z velocity standard deviation. (m/s)"; LPE_GPS_XY "LPE_GPS_XY - Minimum GPS xy standard deviation, uses reported EPH if greater. (m)"; LPE_GPS_Z "LPE_GPS_Z - Minimum GPS z standard deviation, uses reported EPV if greater. (m)"; LPE_LAND_VXY "LPE_LAND_VXY - Land detector xy velocity standard deviation (m/s)"; LPE_LAND_Z "LPE_LAND_Z - Land detector z standard deviation (m)"; LPE_LAT "LPE_LAT - Local origin latitude for nav w/o GPS (deg)"; LPE_LDR_OFF_Z "LPE_LDR_OFF_Z - Lidar z offset from center of vehicle +down (m)"; LPE_LDR_Z "LPE_LDR_Z - Lidar z standard deviation. (m)"; LPE_LON "LPE_LON - Local origin longitude for nav w/o GPS (deg)"; LPE_PN_B "LPE_PN_B - Accel bias propagation noise density ((m/s^2)/s/sqrt(Hz))"; LPE_PN_P "LPE_PN_P - Position propagation noise density (m/s/sqrt(Hz))"; LPE_PN_T "LPE_PN_T - Terrain random walk noise density, hilly/outdoor (0.1), flat/Indoor (0.001) ((m/s)/(sqrt(hz)))"; LPE_PN_V "LPE_PN_V - Velocity propagation noise density ((m/s)/s/sqrt(Hz))"; LPE_SNR_OFF_Z "LPE_SNR_OFF_Z - Sonar z offset from center of vehicle +down (m)"; LPE_SNR_Z "LPE_SNR_Z - Sonar z standard deviation. (m)"; LPE_T_MAX_GRADE "LPE_T_MAX_GRADE - Terrain maximum percent grade, hilly/outdoor (100 = 45 deg), flat/Indoor (0 = 0 deg) (%)"; LPE_VIC_P "LPE_VIC_P - Vicon position standard deviation. (m)"; LPE_VIS_DELAY "LPE_VIS_DELAY - Vision delay compensaton. (sec)"; LPE_VIS_XY "LPE_VIS_XY - Vision xy standard deviation. (m)"; LPE_VIS_Z "LPE_VIS_Z - Vision z standard deviation. (m)"; LPE_VXY_PUB "LPE_VXY_PUB - Required velocity xy standard deviation to publish position (m/s)"; LPE_X_LP "LPE_X_LP - Cut frequency for state publication (Hz)"; LPE_Z_PUB "LPE_Z_PUB - Required z standard deviation to publish altitude/ terrain (m)"; LPE_FUSION "LPE_FUSION - Integer bitmask controlling data fusion (-)"; Barometer "Use Barometer"; GPS "Use GPS"; LIDAR "Use LIDAR"; Flow "Use Flow"; Sonar "Use Sonar"; Vision "Use Vision"; Mocap "Use Mocap"; Land "Use Land"
      mask Callback Barometer:
      | status = get_param( gcb, 'Barometer' );
      | if strcmp( status, 'on' )
      | 	lpe = bitor( uint8(str2num(get_param( gcb, 'LPE_FUSION' ))), uint8(2^0) );
      | 	set_param( gcb, 'LPE_FUSION', num2str(lpe) );
      | else
      | 	lpe = bitand( uint8(str2num(get_param( gcb, 'LPE_FUSION' ))), bitcmp(uint8(2^0), 'uint8' ));
      | 	set_param( gcb, 'LPE_FUSION', num2str(lpe) );
      | end
      mask Callback GPS:
      | status = get_param( gcb, 'GPS' );
      | if strcmp( status, 'on' )
      | 	lpe = bitor( uint8(str2num(get_param( gcb, 'LPE_FUSION' ))), uint8(2^1) );
      | 	set_param( gcb, 'LPE_FUSION', num2str(lpe) );
      | else
      | 	lpe = bitand( uint8(str2num(get_param( gcb, 'LPE_FUSION' ))), bitcmp(uint8(2^1), 'uint8' ));
      | 	set_param( gcb, 'LPE_FUSION', num2str(lpe) );
      | end
      mask Callback LIDAR:
      | status = get_param( gcb, 'LIDAR' );
      | if strcmp( status, 'on' )
      | 	lpe = bitor( uint8(str2num(get_param( gcb, 'LPE_FUSION' ))), uint8(2^2) );
      | 	set_param( gcb, 'LPE_FUSION', num2str(lpe) );
      | else
      | 	lpe = bitand( uint8(str2num(get_param( gcb, 'LPE_FUSION' ))), bitcmp(uint8(2^2), 'uint8' ));
      | 	set_param( gcb, 'LPE_FUSION', num2str(lpe) );
      | end
      mask Callback Flow:
      | status = get_param( gcb, 'Flow' );
      | if strcmp( status, 'on' )
      | 	lpe = bitor( uint8(str2num(get_param( gcb, 'LPE_FUSION' ))), uint8(2^3) );
      | 	set_param( gcb, 'LPE_FUSION', num2str(lpe) );
      | else
      | 	lpe = bitand( uint8(str2num(get_param( gcb, 'LPE_FUSION' ))), bitcmp(uint8(2^3), 'uint8' ));
      | 	set_param( gcb, 'LPE_FUSION', num2str(lpe) );
      | end
      mask Callback Sonar:
      | status = get_param( gcb, 'Sonar' );
      | if strcmp( status, 'on' )
      | 	lpe = bitor( uint8(str2num(get_param( gcb, 'LPE_FUSION' ))), uint8(2^4) );
      | 	set_param( gcb, 'LPE_FUSION', num2str(lpe) );
      | else
      | 	lpe = bitand( uint8(str2num(get_param( gcb, 'LPE_FUSION' ))), bitcmp(uint8(2^4), 'uint8' ));
      | 	set_param( gcb, 'LPE_FUSION', num2str(lpe) );
      | end
      mask Callback Vision:
      | status = get_param( gcb, 'Vision' );
      | if strcmp( status, 'on' )
      | 	lpe = bitor( uint8(str2num(get_param( gcb, 'LPE_FUSION' ))), uint8(2^5) );
      | 	set_param( gcb, 'LPE_FUSION', num2str(lpe) );
      | else
      | 	lpe = bitand( uint8(str2num(get_param( gcb, 'LPE_FUSION' ))), bitcmp(uint8(2^5), 'uint8' ));
      | 	set_param( gcb, 'LPE_FUSION', num2str(lpe) );
      | end
      mask Callback Mocap:
      | status = get_param( gcb, 'Mocap' );
      | if strcmp( status, 'on' )
      | 	lpe = bitor( uint8(str2num(get_param( gcb, 'LPE_FUSION' ))), uint8(2^6) );
      | 	set_param( gcb, 'LPE_FUSION', num2str(lpe) );
      | else
      | 	lpe = bitand( uint8(str2num(get_param( gcb, 'LPE_FUSION' ))), bitcmp(uint8(2^6), 'uint8' ));
      | 	set_param( gcb, 'LPE_FUSION', num2str(lpe) );
      | end
      mask Callback Land:
      | status = get_param( gcb, 'Land' );
      | if strcmp( status, 'on' )
      | 	lpe = bitor( uint8(str2num(get_param( gcb, 'LPE_FUSION' ))), uint8(2^7) );
      | 	set_param( gcb, 'LPE_FUSION', num2str(lpe) );
      | else
      | 	lpe = bitand( uint8(str2num(get_param( gcb, 'LPE_FUSION' ))), bitcmp(uint8(2^7), 'uint8' ));
      | 	set_param( gcb, 'LPE_FUSION', num2str(lpe) );
      | end
  VBodyMeasured : Outport  Unit=m/s
  VBodyDotMeasured : Outport  Port=2  Unit=m/s^2
  nuBodyMeasured : Outport  Port=3  Unit=rad/s
  nuBodyDotMeasured : Outport  Port=4  Unit=rad/s^2
  xiMeasured : Outport  Port=5  Unit=m
  xiDotMeasured : Outport  Port=6  Unit=m/s
  xiDDotMeasured : Outport  Port=7  Unit=m/s^2
  etaMeasured : Outport  Port=8  Unit=rad
  etaDotMeasured : Outport  Port=9  Unit=rad/s
  etaDDotMeasured : Outport  Port=10  Unit=rad/s^2
  qMeasured : Outport  Port=11
  qDotMeasured : Outport  Port=12
  qDDotMeasured : Outport  Port=13
  gyro : Outport  Port=14
  wires:
  xiDot/1 -> [xiDot]
  xi/1 -> [xi]
  nuBodyDot/1 -> nuBodyDotMeasured/1
  nuBody/1 -> [nuBody]
  VBodyDot/1 -> [VBodyDot], VBodyDotMeasured/1
  VBody/1 -> VBodyMeasured/1
  eta/1 -> etaMeasured/1
  etaDot/1 -> etaDotMeasured/1
  etaDDot/1 -> etaDDotMeasured/1
  q/1 -> [q]
  qDot/1 -> qDotMeasured/1
  qDDot/1 -> qDDotMeasured/1
  [att_q] -> local_position_estimator/2(att_q)
  [mocap_x] -> local_position_estimator/5(mocap_x)
  [mocap_z] -> local_position_estimator/7(mocap_z)
  local_position_estimator/10(lpos_x) -> Mux16/1
  local_position_estimator/11(lpos_y) -> Mux16/2
  local_position_estimator/12(lpos_z) -> Mux16/3
  Demux5/2 -> Scope2/2
  Demux5/1 -> Scope2/1
  Demux5/3 -> Scope2/3
  Demux5/4 -> Scope3/1
  Demux5/5 -> Scope3/2
  Demux5/6 -> Scope3/3
  Demux5/7 -> Scope4/1
  Demux5/8 -> Scope4/2
  Demux5/9 -> Scope4/3
  Demux5/10 -> Scope5/1
  [lpe_states] -> Demux6/1
  Demux6/2 -> Scope6/2
  Demux6/1 -> Scope6/1
  Demux6/3 -> Scope6/3
  Demux6/4 -> Scope7/1
  Demux6/5 -> Scope7/2
  Demux6/6 -> Scope7/3
  Demux6/7 -> Scope8/1
  Demux6/8 -> Scope8/2
  Demux6/9 -> Scope8/3
  Demux6/10 -> Scope9/1
  Constant1/1 -> local_position_estimator/4(mocap_updated)
  [lpe_health] -> Health flag/1
  Constant/1 -> local_position_estimator/1(armed_armed)
  [mocap_ts] -> local_position_estimator/3(mocap_timestamp)
  [xiDot] -> Demux7/1
  Time/1 -> Gain1/1
  [accelero_tsr] -> attitude_estimator_q/15(sensors_sub_accelerometer_timestamp_relative)
  Global reprojection/1(lat) -> attitude_estimator_q/4(global_pos_sub_lat)
  Global reprojection/2(lon) -> attitude_estimator_q/5(global_pos_sub_lon)
  [xi] -> Selector/1
  Selector/1 -> Demux8/1
  Demux8/1 -> Global reprojection/1(x)
  Demux8/2 -> Global reprojection/2(y)
  [att_q] -> Select 8/1, Select 7/1, Select 6/1, Select 5/1
  [q] -> Select 2/1, Select 3/1, Select 4/1, Select 1/1
  Mux6/1 -> Attitude (quaternion)/1
  Mux7/1 -> Attitude (quaternion)/2
  Mux8/1 -> Attitude (quaternion)/3
  Mux9/1 -> Attitude (quaternion)/4
  Select 4/1 -> Mux9/1  "actual4"
  Select 8/1 -> Mux9/2  "est4"
  Select 3/1 -> Mux8/1  "actual3"
  Select 7/1 -> Mux8/2  "est3"
  Select 6/1 -> Mux7/2  "est2"
  Select 2/1 -> Mux7/1  "actual2"
  Select 5/1 -> Mux6/2  "est1"
  Select 1/1 -> Mux6/1  "actual1"
  Constant6/1 -> attitude_estimator_q/3(global_pos_sub_eph)
  [q] -> Magnetometer/1(q)
  Mux10/1 -> "Attitude (roll, pitch, yaw)"/1
  Mux11/1 -> "Attitude (roll, pitch, yaw)"/2
  Mux12/1 -> Mux27/2, "Attitude (roll, pitch, yaw)"/3
  Select 11/1 -> Mux12/1  "actual3"
  Select 14/1 -> Mux12/2  "est3"
  Select 13/1 -> Mux11/2  "est2"
  Select 10/1 -> Mux11/1  "actual2"
  Select 12/1 -> Mux10/2  "est1"
  Select 9/1 -> Mux10/1  "actual1"
  [q] -> Quaternion to Euler Angles1/1
  Quaternion to Euler Angles1/1 -> Radians to Degrees/1  "rpy"
  Quaternion to Euler Angles/1 -> Radians to Degrees1/1  "rpyEst"
  Mux13/1 -> Angular vel/1
  Mux14/1 -> Angular vel/2
  Mux15/1 -> Angular vel/3
  Select 17/1 -> Mux13/1
  Select 15/1 -> Mux14/1
  Select 16/1 -> Mux15/1
  [nuBody] -> Select 17/1, Select 16/1, Select 15/1
  Demux7/2 -> attitude_estimator_q/8(global_pos_sub_vel_e)
  [accelero] -> attitude_estimator_q/14(sensors_sub_accelerometer_m_s2)
  [sensor_ts] -> attitude_estimator_q/12(sensors_sub_timestamp)
  [magneto_ga] -> attitude_estimator_q/16(sensors_sub_magnetometer_ga)
  [nuBody] -> Gyroscope/1(nuBody)
  [gyro] -> attitude_estimator_q/13(sensors_sub_gyro_rad)
  [q] -> Accelerometer/1(q)
  [xiDDot] -> Accelerometer/2(xiDDot)
  Accelerometer/1(accelerometer_m_s2) -> [accelero]
  Accelerometer/2(timestamp_relative) -> [accelero_tsr]
  [mocap_q] -> attitude_estimator_q/10(mocap_sub_q)
  [mocap_ts] -> attitude_estimator_q/11(mocap_sub_timestamp)
  Gain1/1 -> Delay3/1, [timestamp]
  [timestamp] -> Mocap System/3(timestamp)
  [q] -> Mocap System/2(q)
  [xi] -> Mocap System/1(xi)
  Constant2/1 -> local_position_estimator/12(sensor_updated)
  [baro_alt] -> local_position_estimator/9(sensor_baro_alt_meter)
  [baro_tsr] -> local_position_estimator/10(sensor_baro_timestamp_relative)
  Mocap System/1(mocap_x) -> [mocap_x]
  Mocap System/2(mocap_y) -> [mocap_y]
  Mocap System/3(mocap_z) -> [mocap_z]
  [mocap_y] -> local_position_estimator/6(mocap_y)
  Mocap System/4(mocap_q) -> [mocap_q]
  Mocap System/5(mocap_timestamp) -> [mocap_ts]
  attitude_estimator_q/5(att_pub_q) -> [att_q]
  Delay3/1 -> [sensor_ts]
  [sensor_ts] -> local_position_estimator/11(sensor_timestamp)
  [xi] -> Barometer/1(xi)
  [timestamp] -> Barometer/2(timestamp)
  Barometer/1(baro_alt_meter) -> [baro_alt]
  Barometer/2(timestamp_relative) -> [baro_tsr]
  Gyroscope/1(gyro_rad) -> gyro/1, [gyro]
  [timestamp] -> Magnetometer/2(timestamp)
  Magnetometer/2(timestamp_relative) -> [magneto_tsr]
  Magnetometer/1(magnetometer_ga) -> [magneto_ga]
  [magneto_tsr] -> attitude_estimator_q/17(sensors_sub_magnetometer_timestamp_relative)
  Demux7/1 -> attitude_estimator_q/7(global_pos_sub_vel_n)
  Demux7/3 -> attitude_estimator_q/9(global_pos_sub_vel_d)
  [sensor_ts] -> attitude_estimator_q/6(global_pos_sub_timestamp)
  Mux16/1 -> [lpe_pos]
  local_position_estimator/7(lpos_vx) -> Mux17/1
  local_position_estimator/8(lpos_vy) -> Mux17/2
  local_position_estimator/9(lpos_vz) -> Mux17/3
  Mux17/1 -> [lpe_vel]
  local_position_estimator/4(gpos_vel_n) -> Mux18/1
  local_position_estimator/5(gpos_vel_e) -> Mux18/2
  local_position_estimator/6(gpos_vel_d) -> Mux18/3
  Mux18/1 -> [gpos_vel]
  local_position_estimator/1(est_status_covariances) -> [lpe_cov]
  local_position_estimator/2(est_status_health_flags) -> [lpe_health]
  local_position_estimator/3(est_status_states) -> [lpe_states]
  [att_q] -> Quaternion to Euler Angles/1
  Mux19/1 -> Position/1
  Mux20/1 -> Position/2
  Mux21/1 -> Position/3
  Select 19/1 -> Mux21/1  "actual3"
  Select 22/1 -> Mux21/2  "est3"
  Select 21/1 -> Mux20/2  "est2"
  Select 18/1 -> Mux20/1  "actual2"
  Select 20/1 -> Mux19/2  "est1"
  Select 23/1 -> Mux19/1  "actual1"
  [lpe_pos] -> To Workspace1/1, Select 20/1, Select 21/1, Select 22/1
  [lpe_cov] -> Demux5/1
  [xi] -> Select 23/1, Select 18/1, Select 19/1, To Workspace/1
  Mux1/1 -> Velocity/1
  Mux2/1 -> Velocity/2
  Mux3/1 -> Velocity/3
  Select 25/1 -> Mux3/1  "actual3"
  Select 28/1 -> Mux3/2  "est3"
  Select 27/1 -> Mux2/2  "est2"
  Select 24/1 -> Mux2/1  "actual2"
  Select 26/1 -> Mux1/2  "est1"
  Select 29/1 -> Mux1/1  "actual1"
  [lpe_vel] -> To Workspace5/1, Select 28/1, Select 27/1, Select 26/1  "velEst"
  [xiDot] -> To Workspace4/1, Select 25/1, Select 24/1, Select 29/1  "vel"
  Mux4/1 -> Velocity (Global)/1
  Mux5/1 -> Velocity (Global)/2
  Mux22/1 -> Velocity (Global)/3
  Select 31/1 -> Mux22/1  "actual3"
  Select 34/1 -> Mux22/2  "est3"
  Select 33/1 -> Mux5/2  "est2"
  Select 30/1 -> Mux5/1  "actual2"
  Select 32/1 -> Mux4/2  "est1"
  Select 35/1 -> Mux4/1  "actual1"
  [gpos_vel] -> Select 32/1, Select 33/1, Select 34/1
  [xiDot] -> Select 35/1, Select 30/1, Select 31/1
  [accelero] -> local_position_estimator/8(sensor_accelerometer_m_s2)
  local_position_estimator/13(lpos_yaw) -> [lpe_yaw]
  Mux/1 -> [att_nuBody]
  attitude_estimator_q/3(att_pub_pitchspeed) -> Mux/2
  attitude_estimator_q/2(att_pub_rollspeed) -> Mux/1
  attitude_estimator_q/4(att_pub_yawspeed) -> Mux/3
  Select 38/1 -> Mux13/2
  Select 37/1 -> Mux15/2
  [att_nuBody] -> Select 38/1, Select 36/1, Select 37/1
  Select 36/1 -> Mux14/2
  Mux23/1 -> [att_xiDDot]
  attitude_estimator_q/7(ctrl_state_pub_y_acc) -> Mux23/2
  attitude_estimator_q/6(ctrl_state_pub_x_acc) -> Mux23/1
  attitude_estimator_q/8(ctrl_state_pub_z_acc) -> Mux23/3
  Mux24/1 -> Acceleration/1
  Mux25/1 -> Acceleration/2
  Mux26/1 -> Acceleration/3
  Select 41/1 -> Mux24/1  "xDDot"
  Select 39/1 -> Mux25/1  "yDDot"
  Select 40/1 -> Mux26/1  "zDDot"
  [accelero] -> Select 39/1, Select 40/1, Select 41/1
  Select 44/1 -> Mux24/2  "xDDotFilt"
  Select 43/1 -> Mux26/2  "zDDotFilt"
  [att_xiDDot] -> Select 43/1, Select 42/1, Select 44/1
  Select 42/1 -> Mux25/2  "yDDotFild"
  attitude_estimator_q/1(att_pub_timestamp) -> [att_timestamp]
  [att_q] -> qMeasured/1
  [att_nuBody] -> nuBodyMeasured/1
  xiDDot/1 -> xiDDotMeasured/1, [xiDDot]
  [lpe_pos] -> xiMeasured/1
  [lpe_vel] -> xiDotMeasured/1
  Ground/1 -> attitude_estimator_q/2(airspeed_sub_timestamp), attitude_estimator_q/1(airspeed_sub_indicated_airspeed_m_s)
  [lpe_yaw] -> Radians to Degrees2/1
  Mux27/1 -> Yaw/1
  Quaternion to Rotation Matrix/1 -> Math Function/1
  Math Function/1 -> Matrix Multiply/1
  [q] -> Quaternion to Rotation Matrix/1
  [xiDDot] -> Matrix Multiply/2
  Matrix Multiply/1 -> Select 46/1, Select 45/1, Select 50/1  "xiDDot_rot"
  [VBodyDot] -> Select 49/1, Select 48/1, Select 47/1  "VBodyDot"
  Mux31/1 -> Acc. comparison/3
  Mux29/1 -> Acc. comparison/1
  Select 46/1 -> Mux31/1  "calc3"
  Select 45/1 -> Mux30/1  "calc2"
  Select 50/1 -> Mux29/1  "calc1"
  Mux30/1 -> Acc. comparison/2
  Select 48/1 -> Mux30/2  "act2"
  Select 49/1 -> Mux31/2  "act3"
  Select 47/1 -> Mux29/2  "act1"
  Accelerometer1/2(timestamp_relative) -> Goto32/1
  Accelerometer1/1(accelerometer_m_s2) -> Goto31/1
  From55/1 -> Accelerometer1/1(q)
  From56/1 -> Accelerometer1/2(VBodyDot)
  Radians to Degrees/1 -> Select 11/1, Select 10/1, Select 9/1
  Radians to Degrees1/1 -> Select 14/1, Select 13/1, Select 12/1
  Radians to Degrees2/1 -> Mux27/1
